simulink model "servo_imu_control"  (R2021b)
settings: Solver=VariableStepAuto  StartTime=0.0  StopTime=50  FixedStep=1e-2  RelTol=1e-3
undefined symbols (not defined in the file): CR, LF
libraries: instrumentseriallib x5, slrealtimeutilitieslib x1, slctrlblks x1, slpidlib x1
settings Model: Creator=eugen  LastModifiedBy=eugen

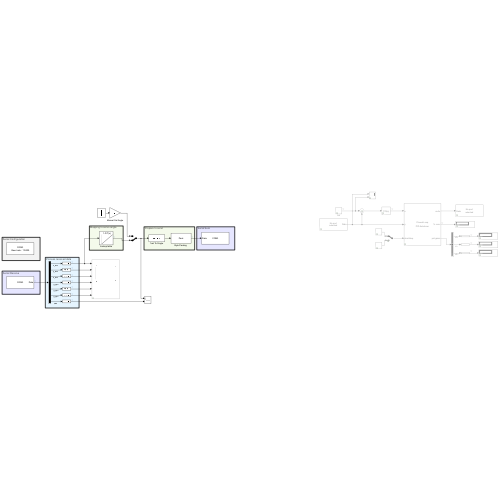
[thumbnail: Simulink's stored preview of the top-level diagram]
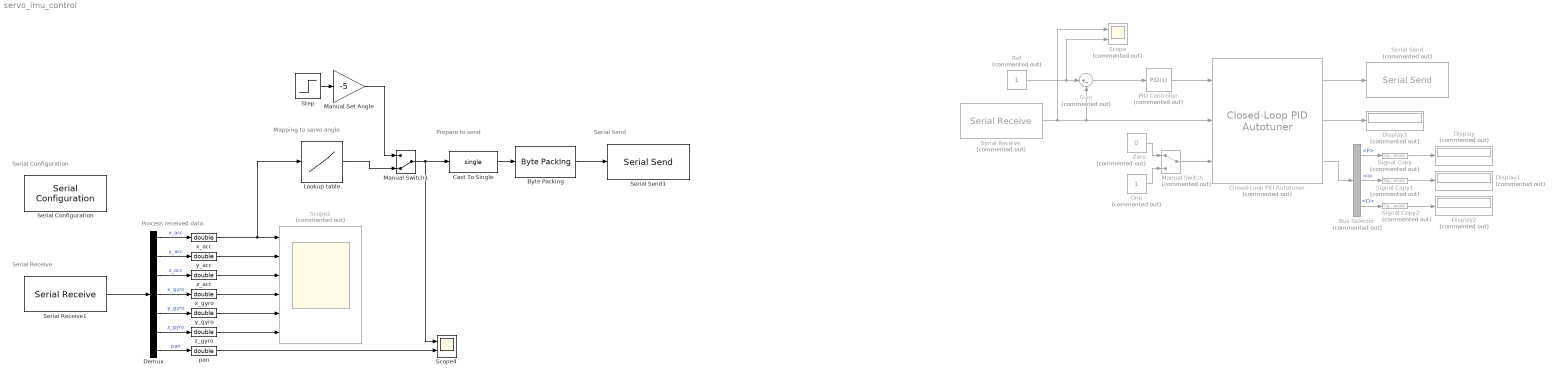
== system servo_imu_control ==
  note: Process received data
  note: Prepare to send
  note: Serial Send
  note: Serial Receive
  note: Mapping to servo angle
  note: Serial Configuration
  Bus Selector : BusSelector  Commented=on  OutputSignals=P,I,D
  "Byte Packing " : slrealtimeutilitieslib/Byte Packing  MaskPackedDataType=uint32  MaskUnpackedDataTypes={'single'}  MaskAlignment=4
  "Cast To Single " : DataTypeConversion  OutDataTypeStr=single
  Closed-Loop PID Autotuner : slctrlblks/Closed-Loop PID Autotuner  Commented=on  PIDType=PID  PIDForm=Parallel  TimeDomain=discrete-time  DiscreteTs=0.02  TuningTs=0.2  UseTuningTs=off  IntegratorFormula=Forward Euler  FilterFormula=Forward Euler  ContinuousTs=0.02  Bandwidth=2*6.28  UseExternalWC=off  TargetPM=60  UseExternalPM=off  UseExternalAchievedPM=off  ExperimentMode=Superposition  PlantType=Stable  PlantSign=Positive  AmpSine=10  UseExternalAmpSine=off  UseExternalFRD=off  UseExternalU0=off  UseCompanion=off  NotDeployTuningModule=off  UsePLCCoder=off  OutputMode=control action + perturbation  BlockDataType=double  UseConnectedPID=on  blockpath=[]  tunedP=0  tunedI=0  tunedD=0  tunedN=100  tunedPM=0  EstimationWindowSize=3  UseExternalTuningParams=off  OutputChoice=VariantCandD  SingleMultiRateVariant=SingleSamplingRate  ExperimentModeVariant=VariantSuperimposed  NumEstimationPeriods=4  NumSettlingPeriods=2
      settings: SourceProductBaseCode=SD
  Demux : Demux  Outputs=7
  Display{,1..3} (4 alike) : Display  Commented=on
  Lookup table : Lookup_n-D  NumberOfTableDimensions=1  BreakpointsForDimension1=[-10000 9000]  Table=[-45 45]  InternalRulePriority=Speed  RndMeth=Simplest  InputSameDT=on
  Manual Set Angle : Gain  Gain=-5
  Manual Switch : ManualSwitch  Commented=on
  Manual Switch1 : ManualSwitch  CurrentSetting=0
  One : Constant  Commented=on  OutDataTypeStr=Inherit: Inherit via back propagation
  PID Controller : slpidlib/PID Controller  Commented=on  Controller=PID  Form=Parallel  TimeDomain=Continuous-time  UseExternalTs=off  SampleTime=-1  IntegratorMethod=Forward Euler  FilterMethod=Forward Euler  ControllerParametersSource=internal  P=1  I=1  D=0  UseFilter=on  N=100  TunerSelectOption=Transfer Function Based (PID Tuner App)  InitialConditionSource=internal  InitialConditionForIntegrator=0  InitialConditionForFilter=0  DifferentiatorICPrevScaledInput=0  ExternalReset=none  TrackingMode=off  Kt=1  LimitOutput=off  SatLimitsSource=internal  UpperSaturationLimit=inf  LowerSaturationLimit=-inf  LinearizeAsGain=on  AntiWindupMode=none  Kb=1  POutMin=[]  POutMax=[]  IOutMin=[]  IOutMax=[]  DOutMin=[]  DOutMax=[]  NOutMin=[]  NOutMax=[]  SumOutMin=[]  SumOutMax=[]  SaturationOutMin=[]  SaturationOutMax=[]  PParamMin=[]  PParamMax=[]  IParamMin=[]  IParamMax=[]  DParamMin=[]  DParamMax=[]  NParamMin=[]  NParamMax=[]  KbParamMin=[]  KbParamMax=[]  KtParamMin=[]  KtParamMax=[]  KbOutMin=[]  KbOutMax=[]  KtOutMin=[]  KtOutMax=[]  IntegratorOutMin=[]  IntegratorOutMax=[]  FilterOutMin=[]  FilterOutMax=[]  SumI1OutMin=[]  SumI1OutMax=[]  SumI2OutMin=[]  SumI2OutMax=[]  SumI3OutMin=[]  SumI3OutMax=[]  SumI4OutMin=[]  SumI4OutMax=[]  SumDOutMin=[]  SumDOutMax=[]  DifferentiatorOutMin=[]  DifferentiatorOutMax=[]  FilterDiffOutCoefMin=[]  FilterDiffOutCoefMax=[]  ReciprocalOutMin=[]  ReciprocalOutMax=[]  SumDenOutMin=[]  SumDenOutMax=[]  SumNumOutMin=[]  SumNumOutMax=[]  DivideOutMin=[]  DivideOutMax=[]  UdiffTsProdOutMin=[]  UdiffTsProdOutMax=[]  NTsProdOutMin=[]  NTsProdOutMax=[]  UintegralTsProdOutMin=[]  UintegralTsProdOutMax=[]  UngainTsProdOutMin=[]  UngainTsProdOutMax=[]  IntegratorContinuousStateAttributes=''  IntegratorStateMustResolveToSignalObject=off  IntegratorRTWStateStorageClass=Auto  FilterContinuousStateAttributes=''  FilterStateMustResolveToSignalObject=off  FilterRTWStateStorageClass=Auto  ParallelPVariant=InternalParameters  IdealPVariant=Disabled  IVariant=InternalParameters  DVariant=InternalParameters  IntegratorVariant=Continuous  SatVariant=Disabled  AWVariant=Passthrough  PCopyVariant=Disabled  TRVariant=Disabled  FdbkBlocksVariant=Forward  IdealPFdbkVariant=Disabled  SatFdbkVariant=Disabled  DerivativeFilterVariant=ContFilter  NVariant=InternalParameters  NCopyVariant=Disabled  FilterICVariant=InternalICsFilter  IntegratorICVariant=InternalICs  ExternalResetVariant=Disabled  TRSumVariant=Passthrough  SumFdbkVariant=Disabled  SumVariant=Sum_PID  TsampFilterVariant=InternalTs  TsampNgainVariant=Passthrough  TsampIntegralVariant=Passthrough  ExternalSaturationOutDataTypeStr=Inherit: Same as second input
  Ref : Constant  Commented=on
  Scope : Scope  Commented=on  NumInputPorts=2
  Scope2 : Scope  Commented=on  NumInputPorts=6
  Scope4 : Scope  NumInputPorts=2
  Serial Configuration : instrumentseriallib/Serial Configuration  Priority=-200000  Port=COM3  ComPort=COM3  BaudRate=115200  DataBits=8  Parity=none  StopBits=1  ByteOrder=little-endian  FlowControl=none  Timeout=10  SimulateUsing=Interpreted execution  BlockInModel=on
  Serial Receive : instrumentseriallib/Serial Receive  Priority=1  Commented=on  Port=<Select a port...>  ComPort=COM5  DataType=single  SaveDataType=uint8  ToggleHeader=on  Header='A'  ToggleTerminator=on  Terminator=LF ('\n')  CustomTerminator=[]  ToggleDataSize=on  DataSize=[1 1]  EnableBlockingMode=on  ActionDataUnavailable=Output last received value  ActionWhenDataUnavailable=Output last received value  CustomValue=0  SampleTime=0.05  SimulateUsing=Interpreted execution  BlockInModel=on
  Serial Receive1 : instrumentseriallib/Serial Receive  Port=COM3  ComPort=COM3  DataType=single  SaveDataType=uint8  ToggleHeader=on  Header='A'  ToggleTerminator=on  Terminator=CR/LF ('\r\n')  CustomTerminator=[]  ToggleDataSize=on  DataSize=[1 7]  EnableBlockingMode=on  ActionDataUnavailable=Output last received value  ActionWhenDataUnavailable=Output last received value  CustomValue=0  SampleTime=0.05  SimulateUsing=Interpreted execution  BlockInModel=on
  Serial Send : instrumentseriallib/Serial Send  Priority=1  Commented=on  Port=<Select a port...>  ComPort=COM5  Header=[]  Terminator=<none>  CustomTerminator=[]  EnableBlockingMode=on  SimulateUsing=Interpreted execution  BlockInModel=on
  Serial Send1 : instrumentseriallib/Serial Send  Port=COM3  ComPort=COM3  Header=[]  Terminator=<none>  CustomTerminator=[]  EnableBlockingMode=on  SimulateUsing=Interpreted execution  BlockInModel=on
  Signal Copy : SignalConversion  Commented=on  OverrideOpt=off
  Signal Copy1 : SignalConversion  Commented=on  OverrideOpt=off
  Signal Copy2 : SignalConversion  Commented=on  OverrideOpt=off
  Step : Step  Before=1  SampleTime=0
  Sum : Sum  Commented=on  Inputs=|+-
  Zero : Constant  Commented=on  Value=0  OutDataTypeStr=Inherit: Inherit via back propagation
  pan : DataTypeConversion  OutDataTypeStr=double
  x_acc : DataTypeConversion  OutDataTypeStr=double
  x_gyro : DataTypeConversion  OutDataTypeStr=double
  y_acc : DataTypeConversion  OutDataTypeStr=double
  y_gyro : DataTypeConversion  OutDataTypeStr=double
  z_acc : DataTypeConversion  OutDataTypeStr=double
  z_gyro : DataTypeConversion  OutDataTypeStr=double
  wires:
  Serial Receive/1 -> Scope/1, Sum/2, Closed-Loop PID Autotuner/2
  Ref/1 -> Scope/2, Sum/1
  Sum/1 -> PID Controller/1
  PID Controller/1 -> Closed-Loop PID Autotuner/1
  Closed-Loop PID Autotuner/1 -> Serial Send/1
  Manual Switch/1 -> Closed-Loop PID Autotuner/3
  Zero/1 -> Manual Switch/1
  One/1 -> Manual Switch/2
  Closed-Loop PID Autotuner/3 -> Bus Selector/1
  Bus Selector/1 -> Signal Copy/1  "<P>"
  Bus Selector/2 -> Signal Copy1/1  "<I>"
  Bus Selector/3 -> Signal Copy2/1  "<D>"
  Signal Copy/1 -> Display/1
  Signal Copy1/1 -> Display1/1
  Signal Copy2/1 -> Display2/1
  Closed-Loop PID Autotuner/2 -> Display3/1
  "Cast To Single "/1 -> "Byte Packing "/1
  Serial Receive1/1 -> Demux/1
  Demux/1 -> x_acc/1  "x_acc"
  Demux/2 -> y_acc/1  "y_acc"
  Demux/3 -> z_acc/1  "z_acc"
  y_acc/1 -> Scope2/2
  x_acc/1 -> Lookup table/1, Scope2/1
  z_acc/1 -> Scope2/3
  "Byte Packing "/1 -> Serial Send1/1
  Step/1 -> Manual Set Angle/1
  Demux/4 -> x_gyro/1  "x_gyro"
  Demux/5 -> y_gyro/1  "y_gyro"
  Demux/6 -> z_gyro/1  "z_gyro"
  Demux/7 -> pan/1  "pan"
  pan/1 -> Scope4/2
  x_gyro/1 -> Scope2/4
  y_gyro/1 -> Scope2/5
  z_gyro/1 -> Scope2/6
  Manual Switch1/1 -> Scope4/1, "Cast To Single "/1
  Manual Set Angle/1 -> Manual Switch1/1
  Lookup table/1 -> Manual Switch1/2
